simulink model "chap04"  (R2021a)
settings: Solver=FixedStepDiscrete  StartTime=0.0  StopTime=30  FixedStep=0.001  RelTol=1e-3
undefined symbols (not defined in the file): DiscIntNeverNeededParam
libraries: simulink x4
(part 2 of 7)

== system chap04/Subsystem/Subsystem2 ==
  In19 : Inport
  Bus Creator : BusCreator  Inputs=3
  Bus Selector : BusSelector  OutputSignals=state(tk).node2.xx,state(tk).node1.xx,state(tk).node4.xx,state(tk).node6.xx,state(tk).node2.vx,state(tk).node1.vx,state(tk).node4.vx,state(tk).node6.vx
  Bus Selector1 : BusSelector  OutputSignals=state(tk).node2.xy,state(tk).node1.xy,state(tk).node4.xy,state(tk).node6.xy,state(tk).node2.vy,state(tk).node1.vy,state(tk).node4.vy,state(tk).node6.vy
  Bus Selector2 : BusSelector  OutputSignals=state(tk).node2.xz,state(tk).node1.xz,state(tk).node4.xz,state(tk).node6.xz,state(tk).node2.vz,state(tk).node1.vz,state(tk).node4.vz,state(tk).node6.vz
  Bus Selector3 : BusSelector  OutputSignals=state(t).node2.vx
  Bus Selector4 : BusSelector  OutputSignals=state(t).node2.vy
  Bus Selector5 : BusSelector  OutputSignals=state(t).node2.vz
  Bus Selector6 : BusSelector  OutputSignals=state(t).node2.vx,state(t).node2.vy,state(t).node2.vz
  Bus Selector7 : BusSelector  OutputSignals=state(t).node2.vx,state(t).node2.vy,state(t).node2.vz
  Bus Selector8 : BusSelector  OutputSignals=control.node2.ux,control.node2.uy,control.node2.uz
  Subsystem1 : Subsystem
  Subsystem10 : Subsystem
  Subsystem12 : Subsystem
  Subsystem2 : Subsystem
  Subsystem3 : Subsystem
  Subsystem4 : Subsystem
      settings: PortSchema="{\"entries\":[{\"content\":{\"sides\":[{\"content\":{\"connectorIds\":[\"In1\",\"In2\",\"In3\"]},\"type\":\"ConnectorPlacement.EquallySpacedRectSide\",\"uuid\":\"3c32f130-2df4-4697-80e9-267a8217898e\"},{\"content\":{\"connectorIds\":[\"Out1\"],\"side\":\"RIGHT\"},\"type\":\"ConnectorPlacement.EquallySpacedRectSide\",\"uuid\":\"840675a7-4714-440f-a6ce-75eff1b2763f\"},{\"content\":{\"connectorIds\":[],\"side\":\"TOP\"},\"type\":\"ConnectorPlacement.EquallySpacedRectSide\",\"uuid\":\"5c23af56-4ec3-4a39-a531-12998a0be3c8\"},{\"content\":{\"connectorIds\":[\"Out2\"],\"side\":\"BOTTOM\"},\"type\":\"ConnectorPlacement.EquallySpacedRectSide\",\"uuid\":\"31d953fb-65a0-42e9-a844-060de010f298\"}]},\"type\":\"ConnectorPlacement.EquallySpacedConnector\",\"uuid\":\"61b27aa3-5880-401e-bae3-4611093a191a\"}],\"packageUris\":[\"http://schema.mathworks.com/mf0/Connector/R2020b\"],\"version\":\"1.0\"}"
  Subsystem6 : Subsystem
  Subsystem7 : Subsystem
      settings: PortSchema="{\"entries\":[{\"content\":{\"sides\":[{\"content\":{\"connectorIds\":[\"In1\",\"In2\",\"In3\"]},\"type\":\"ConnectorPlacement.EquallySpacedRectSide\",\"uuid\":\"3c32f130-2df4-4697-80e9-267a8217898e\"},{\"content\":{\"connectorIds\":[\"Out1\"],\"side\":\"RIGHT\"},\"type\":\"ConnectorPlacement.EquallySpacedRectSide\",\"uuid\":\"840675a7-4714-440f-a6ce-75eff1b2763f\"},{\"content\":{\"connectorIds\":[],\"side\":\"TOP\"},\"type\":\"ConnectorPlacement.EquallySpacedRectSide\",\"uuid\":\"5c23af56-4ec3-4a39-a531-12998a0be3c8\"},{\"content\":{\"connectorIds\":[\"Out2\"],\"side\":\"BOTTOM\"},\"type\":\"ConnectorPlacement.EquallySpacedRectSide\",\"uuid\":\"31d953fb-65a0-42e9-a844-060de010f298\"}]},\"type\":\"ConnectorPlacement.EquallySpacedConnector\",\"uuid\":\"61b27aa3-5880-401e-bae3-4611093a191a\"}],\"packageUris\":[\"http://schema.mathworks.com/mf0/Connector/R2020b\"],\"version\":\"1.0\"}"
  Subsystem8 : Subsystem
      settings: PortSchema="{\"entries\":[{\"content\":{\"sides\":[{\"content\":{\"connectorIds\":[\"In1\",\"In2\",\"In3\"]},\"type\":\"ConnectorPlacement.EquallySpacedRectSide\",\"uuid\":\"3c32f130-2df4-4697-80e9-267a8217898e\"},{\"content\":{\"connectorIds\":[\"Out1\"],\"side\":\"RIGHT\"},\"type\":\"ConnectorPlacement.EquallySpacedRectSide\",\"uuid\":\"840675a7-4714-440f-a6ce-75eff1b2763f\"},{\"content\":{\"connectorIds\":[],\"side\":\"TOP\"},\"type\":\"ConnectorPlacement.EquallySpacedRectSide\",\"uuid\":\"5c23af56-4ec3-4a39-a531-12998a0be3c8\"},{\"content\":{\"connectorIds\":[\"Out2\"],\"side\":\"BOTTOM\"},\"type\":\"ConnectorPlacement.EquallySpacedRectSide\",\"uuid\":\"31d953fb-65a0-42e9-a844-060de010f298\"}]},\"type\":\"ConnectorPlacement.EquallySpacedConnector\",\"uuid\":\"61b27aa3-5880-401e-bae3-4611093a191a\"}],\"packageUris\":[\"http://schema.mathworks.com/mf0/Connector/R2020b\"],\"version\":\"1.0\"}"
  u2 : Outport
  wires:
  Bus Creator/1 -> u2/1  "node2"
  Bus Selector6/1 -> Subsystem12/4(vx)  "<vx>"
  Bus Selector6/2 -> Subsystem12/5(vy)  "<vy>"
  Bus Selector6/3 -> Subsystem12/6(vz)  "<vz>"
  [Sz] -> Subsystem12/3(Sz)
  [Sx] -> Subsystem12/1(Sx)
  [state] -> Bus Selector6/1
  [Sy] -> Subsystem12/2(Sy)
  Subsystem12/1(" gain") -> [gain]
  Subsystem10/1(ux) -> Bus Creator/1  "ux"
  Subsystem10/2(uy) -> Bus Creator/2  "uy"
  Subsystem10/3(uz) -> Bus Creator/3  "uz"
  Bus Selector8/3 -> Subsystem3/8(uz)  "<uz>"
  Bus Selector7/3 -> Subsystem3/4(vz)  "<vz>"
  Bus Selector7/2 -> Subsystem3/3(vy)  "<vy>"
  Bus Selector7/1 -> Subsystem3/2(vx)  "<vx>"
  Bus Selector8/1 -> Subsystem3/6(ux)  "<ux>"
  [state] -> Bus Selector7/1
  Bus Selector8/2 -> Subsystem3/7(uy)  "<uy>"
  [state] -> Bus Selector8/1
  Subsystem3/1(xdut1) -> Subsystem10/1(utx)
  Subsystem3/2(ydut1) -> Subsystem10/2(uty)
  Subsystem3/3(zdut1) -> Subsystem10/3(utz)
  Subsystem8/2(Sz) -> [Sz]
  Subsystem7/1(ux) -> Subsystem3/5(uty)
  Subsystem1/1(p2y) -> Subsystem7/2(uty)
  [state] -> Bus Selector4/1
  Subsystem4/1(ux) -> Subsystem3/1(utx)
  Subsystem2/1(p2z) -> Subsystem8/2(utz)
  Bus Selector4/1 -> Subsystem7/1(vy1)  "<vy>"
  Bus Selector5/1 -> Subsystem8/1(vz1)  "<vz>"
  [gain] -> Subsystem8/3(gain)
  [gain] -> Subsystem4/3(gain)
  Subsystem8/1(ux) -> Subsystem3/9(utz)
  [gain] -> Subsystem7/3(gain)
  [state] -> Bus Selector3/1
  Subsystem6/1(p2x) -> Subsystem4/2(utx)
  Subsystem7/2(Sy) -> [Sy]
  Bus Selector3/1 -> Subsystem4/1(vx1)  "<vx>"
  Subsystem4/2(Sx) -> [Sx]
  [state] -> Bus Selector5/1
  In19/1 -> [state], Bus Selector2/1, Bus Selector/1, Bus Selector1/1
  Bus Selector1/6 -> Subsystem1/6(vy1)  "<vy>"
  Bus Selector2/6 -> Subsystem2/6(vz1)  "<vz>"
  Bus Selector/7 -> Subsystem6/7(vx4)  "<vx>"
  Bus Selector/3 -> Subsystem6/3(xx4)  "<xx>"
  Bus Selector1/2 -> Subsystem1/2(xy1)  "<xy>"
  Bus Selector1/5 -> Subsystem1/5(vy2)  "<vy>"
  Bus Selector/2 -> Subsystem6/2(xx1)  "<xx>"
  Bus Selector/6 -> Subsystem6/6(vx1)  "<vx>"
  Bus Selector/8 -> Subsystem6/8(vx6)  "<vx>"
  Bus Selector1/8 -> Subsystem1/8(vy6)  "<vy>"
  Bus Selector/1 -> Subsystem6/1(xx2)  "<xx>"
  Bus Selector/5 -> Subsystem6/5(vx2)  "<vx>"
  Bus Selector1/1 -> Subsystem1/1(xy2)  "<xy>"
  Bus Selector2/3 -> Subsystem2/3(xz4)  "<xz>"
  Bus Selector2/4 -> Subsystem2/4(xz6)  "<xz>"
  Bus Selector2/5 -> Subsystem2/5(vz2)  "<vz>"
  Bus Selector2/7 -> Subsystem2/7(vz4)  "<vz>"
  Bus Selector2/1 -> Subsystem2/1(xz2)  "<xz>"
  Bus Selector2/2 -> Subsystem2/2(xz1)  "<xz>"
  Bus Selector1/7 -> Subsystem1/7(vy4)  "<vy>"
  Bus Selector1/3 -> Subsystem1/3(xy4)  "<xy>"
  Bus Selector1/4 -> Subsystem1/4(xy6)  "<xy>"
  Bus Selector/4 -> Subsystem6/4(xx6)  "<xx>"
  Bus Selector2/8 -> Subsystem2/8(vz6)  "<vz>"

== system chap04/Subsystem/Subsystem3 ==
  In19 : Inport
  Bus Creator : BusCreator  Inputs=3
  Bus Selector : BusSelector  OutputSignals=state(tk).node4.xx,state(tk).node2.xx,state(tk).node3.xx,state(tk).node5.xx,state(tk).node4.vx,state(tk).node2.vx,state(tk).node3.vx,state(tk).node5.vx
  Bus Selector1 : BusSelector  OutputSignals=state(tk).node4.xy,state(tk).node2.xy,state(tk).node3.xy,state(tk).node5.xy,state(tk).node4.vy,state(tk).node2.vy,state(tk).node3.vy,state(tk).node5.vy
  Bus Selector2 : BusSelector  OutputSignals=state(tk).node4.xz,state(tk).node2.xz,state(tk).node3.xz,state(tk).node5.xz,state(tk).node4.vz,state(tk).node2.vz,state(tk).node3.vz,state(tk).node5.vz
  Bus Selector3 : BusSelector  OutputSignals=state(t).node4.vx
  Bus Selector4 : BusSelector  OutputSignals=state(t).node4.vy
  Bus Selector5 : BusSelector  OutputSignals=state(t).node4.vz
  Bus Selector6 : BusSelector  OutputSignals=state(t).node4.vx,state(t).node4.vy,state(t).node4.vz
  Bus Selector7 : BusSelector  OutputSignals=state(t).node4.vx,state(t).node4.vy,state(t).node4.vz
  Bus Selector8 : BusSelector  OutputSignals=control.node4.ux,control.node4.uy,control.node4.uz
  Subsystem1 : Subsystem
  Subsystem10 : Subsystem
  Subsystem12 : Subsystem
  Subsystem2 : Subsystem
  Subsystem3 : Subsystem
  Subsystem4 : Subsystem
      settings: PortSchema="{\"entries\":[{\"content\":{\"sides\":[{\"content\":{\"connectorIds\":[\"In1\",\"In2\",\"In3\"]},\"type\":\"ConnectorPlacement.EquallySpacedRectSide\",\"uuid\":\"3c32f130-2df4-4697-80e9-267a8217898e\"},{\"content\":{\"connectorIds\":[\"Out1\"],\"side\":\"RIGHT\"},\"type\":\"ConnectorPlacement.EquallySpacedRectSide\",\"uuid\":\"840675a7-4714-440f-a6ce-75eff1b2763f\"},{\"content\":{\"connectorIds\":[],\"side\":\"TOP\"},\"type\":\"ConnectorPlacement.EquallySpacedRectSide\",\"uuid\":\"5c23af56-4ec3-4a39-a531-12998a0be3c8\"},{\"content\":{\"connectorIds\":[\"Out2\"],\"side\":\"BOTTOM\"},\"type\":\"ConnectorPlacement.EquallySpacedRectSide\",\"uuid\":\"31d953fb-65a0-42e9-a844-060de010f298\"}]},\"type\":\"ConnectorPlacement.EquallySpacedConnector\",\"uuid\":\"61b27aa3-5880-401e-bae3-4611093a191a\"}],\"packageUris\":[\"http://schema.mathworks.com/mf0/Connector/R2020b\"],\"version\":\"1.0\"}"
  Subsystem6 : Subsystem
  Subsystem7 : Subsystem
      settings: PortSchema="{\"entries\":[{\"content\":{\"sides\":[{\"content\":{\"connectorIds\":[\"In1\",\"In2\",\"In3\"]},\"type\":\"ConnectorPlacement.EquallySpacedRectSide\",\"uuid\":\"3c32f130-2df4-4697-80e9-267a8217898e\"},{\"content\":{\"connectorIds\":[\"Out1\"],\"side\":\"RIGHT\"},\"type\":\"ConnectorPlacement.EquallySpacedRectSide\",\"uuid\":\"840675a7-4714-440f-a6ce-75eff1b2763f\"},{\"content\":{\"connectorIds\":[],\"side\":\"TOP\"},\"type\":\"ConnectorPlacement.EquallySpacedRectSide\",\"uuid\":\"5c23af56-4ec3-4a39-a531-12998a0be3c8\"},{\"content\":{\"connectorIds\":[\"Out2\"],\"side\":\"BOTTOM\"},\"type\":\"ConnectorPlacement.EquallySpacedRectSide\",\"uuid\":\"31d953fb-65a0-42e9-a844-060de010f298\"}]},\"type\":\"ConnectorPlacement.EquallySpacedConnector\",\"uuid\":\"61b27aa3-5880-401e-bae3-4611093a191a\"}],\"packageUris\":[\"http://schema.mathworks.com/mf0/Connector/R2020b\"],\"version\":\"1.0\"}"
  Subsystem8 : Subsystem
      settings: PortSchema="{\"entries\":[{\"content\":{\"sides\":[{\"content\":{\"connectorIds\":[\"In1\",\"In2\",\"In3\"]},\"type\":\"ConnectorPlacement.EquallySpacedRectSide\",\"uuid\":\"3c32f130-2df4-4697-80e9-267a8217898e\"},{\"content\":{\"connectorIds\":[\"Out1\"],\"side\":\"RIGHT\"},\"type\":\"ConnectorPlacement.EquallySpacedRectSide\",\"uuid\":\"840675a7-4714-440f-a6ce-75eff1b2763f\"},{\"content\":{\"connectorIds\":[],\"side\":\"TOP\"},\"type\":\"ConnectorPlacement.EquallySpacedRectSide\",\"uuid\":\"5c23af56-4ec3-4a39-a531-12998a0be3c8\"},{\"content\":{\"connectorIds\":[\"Out2\"],\"side\":\"BOTTOM\"},\"type\":\"ConnectorPlacement.EquallySpacedRectSide\",\"uuid\":\"31d953fb-65a0-42e9-a844-060de010f298\"}]},\"type\":\"ConnectorPlacement.EquallySpacedConnector\",\"uuid\":\"61b27aa3-5880-401e-bae3-4611093a191a\"}],\"packageUris\":[\"http://schema.mathworks.com/mf0/Connector/R2020b\"],\"version\":\"1.0\"}"
  u4 : Outport
  wires:
  Bus Creator/1 -> u4/1  "node4"
  Bus Selector/2 -> Subsystem6/2(xx2)  "<xx>"
  Bus Selector1/7 -> Subsystem1/7(vy3)  "<vy>"
  Bus Selector1/4 -> Subsystem1/4(xy5)  "<xy>"
  Bus Selector2/3 -> Subsystem2/3(xz3)  "<xz>"
  Bus Selector/8 -> Subsystem6/8(vx5)  "<vx>"
  Bus Selector2/2 -> Subsystem2/2(xx2)  "<xz>"
  Bus Selector2/4 -> Subsystem2/4(xz5)  "<xz>"
  Bus Selector1/5 -> Subsystem1/5(vy4)  "<vy>"
  Bus Selector1/2 -> Subsystem1/2(xy2)  "<xy>"
  Bus Selector2/7 -> Subsystem2/7(vz3)  "<vz>"
  Bus Selector2/5 -> Subsystem2/5(vz4)  "<vz>"
  Bus Selector1/6 -> Subsystem1/6(vy2)  "<vy>"
  Bus Selector2/8 -> Subsystem2/8(vz5)  "<vz>"
  Bus Selector2/6 -> Subsystem2/6(vz2)  "<vz>"
  Bus Selector1/3 -> Subsystem1/3(xy3)  "<xy>"
  Bus Selector2/1 -> Subsystem2/1(xz4)  "<xz>"
  Bus Selector/5 -> Subsystem6/5(vx4)  "<vx>"
  Bus Selector/1 -> Subsystem6/1(xx4)  "<xx>"
  Bus Selector/3 -> Subsystem6/3(xx3)  "<xx>"
  Bus Selector1/8 -> Subsystem1/8(vy5)  "<vy>"
  Bus Selector1/1 -> Subsystem1/1(xy4)  "<xy>"
  Bus Selector/7 -> Subsystem6/7(vx3)  "<vx>"
  Bus Selector/6 -> Subsystem6/6(vx2)  "<vx>"
  Bus Selector/4 -> Subsystem6/4(xx5)  "<xx>"
  [state] -> Bus Selector5/1
  Subsystem2/1(utx) -> Subsystem8/2(utz)
  Bus Selector5/1 -> Subsystem8/1(vz4)  "<vz>"
  [state] -> Bus Selector4/1
  [gain] -> Subsystem8/3(gain)
  Bus Selector6/3 -> Subsystem12/6(vz)  "<vz>"
  Bus Selector6/1 -> Subsystem12/4(vx)  "<vx>"
  [Sx] -> Subsystem12/1(Sx)
  [Sz] -> Subsystem12/3(Sz)
  Subsystem12/1(" gain") -> [gain]
  Subsystem6/1(utx) -> Subsystem4/2(utx)
  In19/1 -> [state], Bus Selector2/1, Bus Selector/1, Bus Selector1/1
  [state] -> Bus Selector6/1
  Bus Selector4/1 -> Subsystem7/1(vy4)  "<vy>"
  Subsystem1/1(utx) -> Subsystem7/2(uty)
  Bus Selector3/1 -> Subsystem4/1(vx4)  "<vx>"
  Subsystem7/2(Sy) -> [Sy]
  [gain] -> Subsystem7/3(gain)
  [Sy] -> Subsystem12/2(Sy)
  [gain] -> Subsystem4/3(gain)
  [state] -> Bus Selector3/1
  Subsystem8/2(Sz) -> [Sz]
  Bus Selector6/2 -> Subsystem12/5(vy)  "<vy>"
  Subsystem4/2(Sx) -> [Sx]
  Subsystem10/1(ux) -> Bus Creator/1  "ux"
  Subsystem10/2(uy) -> Bus Creator/2  "uy"
  Subsystem10/3(uz) -> Bus Creator/3  "uz"
  Subsystem4/1(ux) -> Subsystem3/1(utx)
  Subsystem7/1(ux) -> Subsystem3/5(uty)
  Subsystem8/1(ux) -> Subsystem3/9(utz)
  [state] -> Bus Selector7/1
  Bus Selector8/1 -> Subsystem3/6(ux)  "<ux>"
  Bus Selector7/2 -> Subsystem3/3(vy)  "<vy>"
  Bus Selector8/2 -> Subsystem3/7(uy)  "<uy>"
  [state] -> Bus Selector8/1
  Bus Selector7/1 -> Subsystem3/2(vx)  "<vx>"
  Bus Selector7/3 -> Subsystem3/4(vz)  "<vz>"
  Bus Selector8/3 -> Subsystem3/8(uz)  "<uz>"
  Subsystem3/1(udtx) -> Subsystem10/1(utx)
  Subsystem3/2(udty) -> Subsystem10/2(uty)
  Subsystem3/3(udtz) -> Subsystem10/3(utz)

== system chap04/Subsystem/Subsystem4 ==
  In19 : Inport
  Bus Creator : BusCreator  Inputs=3
  Bus Selector : BusSelector  OutputSignals=state(tk).node6.xx,state(tk).node6.xx0,state(tk).node1.xx,state(tk).node2.xx,state(tk).node6.vx,state(tk).node6.vx0,state(tk).node1.vx,state(tk).node2.vx
  Bus Selector1 : BusSelector  OutputSignals=state(tk).node6.xy,state(tk).node6.xy0,state(tk).node1.xy,state(tk).node2.xy,state(tk).node6.vy,state(tk).node6.vy0,state(tk).node1.vy,state(tk).node2.vy
  Bus Selector2 : BusSelector  OutputSignals=state(tk).node6.xz,state(tk).node6.xz0,state(tk).node1.xz,state(tk).node2.xz,state(tk).node6.vz,state(tk).node6.vz0,state(tk).node1.vz,state(tk).node2.vz
  Bus Selector3 : BusSelector  OutputSignals=state(t).node6.vx,state(t).node0.vx
  Bus Selector4 : BusSelector  OutputSignals=state(t).node6.vy,state(t).node0.vx
  Bus Selector5 : BusSelector  OutputSignals=state(t).node6.vz,state(t).node0.vz
  Bus Selector6 : BusSelector  OutputSignals=state(t).node6.vx,state(t).node6.vy,state(t).node6.vz
  Bus Selector7 : BusSelector  OutputSignals=state(t).node6.vx,state(t).node6.vy,state(t).node6.vz
  Bus Selector8 : BusSelector  OutputSignals=control.node6.ux,control.node6.uy,control.node6.uz
  Subsystem1 : Subsystem
  Subsystem10 : Subsystem
  Subsystem12 : Subsystem
  Subsystem2 : Subsystem
  Subsystem3 : Subsystem
  Subsystem4 : Subsystem
      settings: PortSchema="{\"entries\":[{\"content\":{\"sides\":[{\"content\":{\"connectorIds\":[\"In1\",\"In2\",\"In3\",\"In4\"]},\"type\":\"ConnectorPlacement.EquallySpacedRectSide\",\"uuid\":\"3c32f130-2df4-4697-80e9-267a8217898e\"},{\"content\":{\"connectorIds\":[\"Out1\"],\"side\":\"RIGHT\"},\"type\":\"ConnectorPlacement.EquallySpacedRectSide\",\"uuid\":\"840675a7-4714-440f-a6ce-75eff1b2763f\"},{\"content\":{\"connectorIds\":[],\"side\":\"TOP\"},\"type\":\"ConnectorPlacement.EquallySpacedRectSide\",\"uuid\":\"5c23af56-4ec3-4a39-a531-12998a0be3c8\"},{\"content\":{\"connectorIds\":[\"Out2\"],\"side\":\"BOTTOM\"},\"type\":\"ConnectorPlacement.EquallySpacedRectSide\",\"uuid\":\"31d953fb-65a0-42e9-a844-060de010f298\"}]},\"type\":\"ConnectorPlacement.EquallySpacedConnector\",\"uuid\":\"61b27aa3-5880-401e-bae3-4611093a191a\"}],\"packageUris\":[\"http://schema.mathworks.com/mf0/Connector/R2020b\"],\"version\":\"1.0\"}"
  Subsystem6 : Subsystem
  Subsystem7 : Subsystem
      settings: PortSchema="{\"entries\":[{\"content\":{\"sides\":[{\"content\":{\"connectorIds\":[\"In1\",\"In2\",\"In3\",\"In4\"]},\"type\":\"ConnectorPlacement.EquallySpacedRectSide\",\"uuid\":\"3c32f130-2df4-4697-80e9-267a8217898e\"},{\"content\":{\"connectorIds\":[\"Out1\"],\"side\":\"RIGHT\"},\"type\":\"ConnectorPlacement.EquallySpacedRectSide\",\"uuid\":\"840675a7-4714-440f-a6ce-75eff1b2763f\"},{\"content\":{\"connectorIds\":[],\"side\":\"TOP\"},\"type\":\"ConnectorPlacement.EquallySpacedRectSide\",\"uuid\":\"5c23af56-4ec3-4a39-a531-12998a0be3c8\"},{\"content\":{\"connectorIds\":[\"Out2\"],\"side\":\"BOTTOM\"},\"type\":\"ConnectorPlacement.EquallySpacedRectSide\",\"uuid\":\"31d953fb-65a0-42e9-a844-060de010f298\"}]},\"type\":\"ConnectorPlacement.EquallySpacedConnector\",\"uuid\":\"61b27aa3-5880-401e-bae3-4611093a191a\"}],\"packageUris\":[\"http://schema.mathworks.com/mf0/Connector/R2020b\"],\"version\":\"1.0\"}"
  Subsystem8 : Subsystem
      settings: PortSchema="{\"entries\":[{\"content\":{\"sides\":[{\"content\":{\"connectorIds\":[\"In1\",\"In2\",\"In3\",\"In4\"]},\"type\":\"ConnectorPlacement.EquallySpacedRectSide\",\"uuid\":\"3c32f130-2df4-4697-80e9-267a8217898e\"},{\"content\":{\"connectorIds\":[\"Out1\"],\"side\":\"RIGHT\"},\"type\":\"ConnectorPlacement.EquallySpacedRectSide\",\"uuid\":\"840675a7-4714-440f-a6ce-75eff1b2763f\"},{\"content\":{\"connectorIds\":[],\"side\":\"TOP\"},\"type\":\"ConnectorPlacement.EquallySpacedRectSide\",\"uuid\":\"5c23af56-4ec3-4a39-a531-12998a0be3c8\"},{\"content\":{\"connectorIds\":[\"Out2\"],\"side\":\"BOTTOM\"},\"type\":\"ConnectorPlacement.EquallySpacedRectSide\",\"uuid\":\"31d953fb-65a0-42e9-a844-060de010f298\"}]},\"type\":\"ConnectorPlacement.EquallySpacedConnector\",\"uuid\":\"61b27aa3-5880-401e-bae3-4611093a191a\"}],\"packageUris\":[\"http://schema.mathworks.com/mf0/Connector/R2020b\"],\"version\":\"1.0\"}"
  u6 : Outport
  wires:
  Bus Creator/1 -> u6/1  "node6"
  Bus Selector/1 -> Subsystem6/1(xx6)  "<xx>"
  Bus Selector/3 -> Subsystem6/3(xx1)  "<xx>"
  Bus Selector/4 -> Subsystem6/4(xx2)  "<xx>"
  Bus Selector6/3 -> Subsystem12/6(vz)  "<vz>"
  Bus Selector6/1 -> Subsystem12/4(vx)  "<vx>"
  [Sx] -> Subsystem12/1(Sx)
  [Sz] -> Subsystem12/3(Sz)
  Subsystem12/1(" gain") -> [gain]
  In19/1 -> [state], Bus Selector2/1, Bus Selector/1, Bus Selector1/1
  [state] -> Bus Selector6/1
  [Sy] -> Subsystem12/2(Sy)
  Bus Selector6/2 -> Subsystem12/5(vy)  "<vy>"
  Subsystem10/3(uz) -> Bus Creator/3  "uz"
  Subsystem10/2(uy) -> Bus Creator/2  "uy"
  Subsystem10/1(ux) -> Bus Creator/1  "ux"
  Bus Selector7/3 -> Subsystem3/4(vz)  "<vz>"
  Bus Selector7/1 -> Subsystem3/2(vx)  "<vx>"
  [state] -> Bus Selector8/1
  Bus Selector8/1 -> Subsystem3/6(ux)  "<ux>"
  Bus Selector8/2 -> Subsystem3/7(uy)  "<uy>"
  Bus Selector7/2 -> Subsystem3/3(vy)  "<vy>"
  [state] -> Bus Selector7/1
  Bus Selector8/3 -> Subsystem3/8(uz)  "<uz>"
  Subsystem3/2(udty) -> Subsystem10/2(uty)
  Subsystem3/1(udtx) -> Subsystem10/1(utx)
  Subsystem3/3(udtz) -> Subsystem10/3(utz)
  Bus Selector/2 -> Subsystem6/2(xx0)  "<xx0>"
  Bus Selector/5 -> Subsystem6/5(vx6)  "<vx>"
  Bus Selector/6 -> Subsystem6/6(vx0)  "<vx0>"
  Bus Selector/7 -> Subsystem6/7(vx1)  "<vx>"
  Bus Selector/8 -> Subsystem6/8(vx2)  "<vx>"
  Bus Selector1/1 -> Subsystem1/1(xx6)  "<xy>"
  Bus Selector1/2 -> Subsystem1/2(xx0)  "<xy0>"
  Bus Selector1/3 -> Subsystem1/3(xx1)  "<xy>"
  Bus Selector1/4 -> Subsystem1/4(xx2)  "<xy>"
  Bus Selector1/5 -> Subsystem1/5(vx6)  "<vy>"
  Bus Selector1/6 -> Subsystem1/6(vx0)  "<vy0>"
  Bus Selector1/7 -> Subsystem1/7(vx1)  "<vy>"
  Bus Selector1/8 -> Subsystem1/8(vx2)  "<vy>"
  Bus Selector2/1 -> Subsystem2/1(xx6)  "<xz>"
  Bus Selector2/2 -> Subsystem2/2(xx0)  "<xz0>"
  Bus Selector2/3 -> Subsystem2/3(xx1)  "<xz>"
  Bus Selector2/4 -> Subsystem2/4(xx2)  "<xz>"
  Bus Selector2/5 -> Subsystem2/5(vx6)  "<vz>"
  Bus Selector2/6 -> Subsystem2/6(vx0)  "<vz0>"
  Bus Selector2/7 -> Subsystem2/7(vx1)  "<vz>"
  Bus Selector2/8 -> Subsystem2/8(vx2)  "<vz>"
  Subsystem4/2(Sx) -> [Sx]
  Bus Selector5/2 -> Subsystem8/2(vz0)  "<vz>"
  Subsystem7/2(Sy) -> [Sy]
  Subsystem8/2(Sz) -> [Sz]
  [gain] -> Subsystem7/4(gain)
  Subsystem1/1(utx) -> Subsystem7/3(uty)
  Subsystem2/1(utx) -> Subsystem8/3(utz)
  [state] -> Bus Selector3/1
  Bus Selector5/1 -> Subsystem8/1(vz6)  "<vz>"
  Bus Selector4/2 -> Subsystem7/2(vy0)  "<vx>"
  [gain] -> Subsystem4/4(gain)
  [state] -> Bus Selector5/1
  Subsystem8/1(ux) -> Subsystem3/9(utz)
  Subsystem6/1(utx) -> Subsystem4/3(utx)
  Subsystem7/1(ux) -> Subsystem3/5(uty)
  Subsystem4/1(ux) -> Subsystem3/1(utx)
  Bus Selector3/1 -> Subsystem4/1(vx6)  "<vx>"
  Bus Selector3/2 -> Subsystem4/2(vx0)  "<vx>"
  [gain] -> Subsystem8/4(gain)
  [state] -> Bus Selector4/1
  Bus Selector4/1 -> Subsystem7/1(vy6)  "<vy>"

== system chap04/Subsystem/Subsystem5 ==
  In19 : Inport
  Bus Creator : BusCreator  Inputs=3
  Bus Selector : BusSelector  OutputSignals=state(tk).node3.xx,state(tk).node1.xx,state(tk).node4.xx,state(tk).node5.xx,state(tk).node3.vx,state(tk).node1.vx,state(tk).node4.vx,state(tk).node5.vx
  Bus Selector1 : BusSelector  OutputSignals=state(tk).node3.xy,state(tk).node1.xy,state(tk).node4.xy,state(tk).node5.xy,state(tk).node3.vy,state(tk).node1.vy,state(tk).node4.vy,state(tk).node5.vy
  Bus Selector2 : BusSelector  OutputSignals=state(tk).node3.xz,state(tk).node1.xz,state(tk).node4.xz,state(tk).node5.xz,state(tk).node3.vz,state(tk).node1.vz,state(tk).node4.vz,state(tk).node5.vz
  Bus Selector3 : BusSelector  OutputSignals=state(t).node3.vx
  Bus Selector4 : BusSelector  OutputSignals=state(t).node3.vy
  Bus Selector5 : BusSelector  OutputSignals=state(t).node3.vz
  Bus Selector6 : BusSelector  OutputSignals=state(t).node3.vx,state(t).node3.vy,state(t).node3.vz
  Bus Selector7 : BusSelector  OutputSignals=state(t).node3.vx,state(t).node3.vy,state(t).node3.vz
  Bus Selector8 : BusSelector  OutputSignals=control.node3.ux,control.node3.uy,control.node3.uz
  Subsystem1 : Subsystem
  Subsystem10 : Subsystem
  Subsystem12 : Subsystem
  Subsystem2 : Subsystem
  Subsystem3 : Subsystem
  Subsystem4 : Subsystem
      settings: PortSchema="{\"entries\":[{\"content\":{\"sides\":[{\"content\":{\"connectorIds\":[\"In1\",\"In2\",\"In3\"]},\"type\":\"ConnectorPlacement.EquallySpacedRectSide\",\"uuid\":\"3c32f130-2df4-4697-80e9-267a8217898e\"},{\"content\":{\"connectorIds\":[\"Out1\"],\"side\":\"RIGHT\"},\"type\":\"ConnectorPlacement.EquallySpacedRectSide\",\"uuid\":\"840675a7-4714-440f-a6ce-75eff1b2763f\"},{\"content\":{\"connectorIds\":[],\"side\":\"TOP\"},\"type\":\"ConnectorPlacement.EquallySpacedRectSide\",\"uuid\":\"5c23af56-4ec3-4a39-a531-12998a0be3c8\"},{\"content\":{\"connectorIds\":[\"Out2\"],\"side\":\"BOTTOM\"},\"type\":\"ConnectorPlacement.EquallySpacedRectSide\",\"uuid\":\"31d953fb-65a0-42e9-a844-060de010f298\"}]},\"type\":\"ConnectorPlacement.EquallySpacedConnector\",\"uuid\":\"61b27aa3-5880-401e-bae3-4611093a191a\"}],\"packageUris\":[\"http://schema.mathworks.com/mf0/Connector/R2020b\"],\"version\":\"1.0\"}"
  Subsystem6 : Subsystem
  Subsystem7 : Subsystem
      settings: PortSchema="{\"entries\":[{\"content\":{\"sides\":[{\"content\":{\"connectorIds\":[\"In1\",\"In2\",\"In3\"]},\"type\":\"ConnectorPlacement.EquallySpacedRectSide\",\"uuid\":\"3c32f130-2df4-4697-80e9-267a8217898e\"},{\"content\":{\"connectorIds\":[\"Out1\"],\"side\":\"RIGHT\"},\"type\":\"ConnectorPlacement.EquallySpacedRectSide\",\"uuid\":\"840675a7-4714-440f-a6ce-75eff1b2763f\"},{\"content\":{\"connectorIds\":[],\"side\":\"TOP\"},\"type\":\"ConnectorPlacement.EquallySpacedRectSide\",\"uuid\":\"5c23af56-4ec3-4a39-a531-12998a0be3c8\"},{\"content\":{\"connectorIds\":[\"Out2\"],\"side\":\"BOTTOM\"},\"type\":\"ConnectorPlacement.EquallySpacedRectSide\",\"uuid\":\"31d953fb-65a0-42e9-a844-060de010f298\"}]},\"type\":\"ConnectorPlacement.EquallySpacedConnector\",\"uuid\":\"61b27aa3-5880-401e-bae3-4611093a191a\"}],\"packageUris\":[\"http://schema.mathworks.com/mf0/Connector/R2020b\"],\"version\":\"1.0\"}"
  Subsystem8 : Subsystem
      settings: PortSchema="{\"entries\":[{\"content\":{\"sides\":[{\"content\":{\"connectorIds\":[\"In1\",\"In2\",\"In3\"]},\"type\":\"ConnectorPlacement.EquallySpacedRectSide\",\"uuid\":\"3c32f130-2df4-4697-80e9-267a8217898e\"},{\"content\":{\"connectorIds\":[\"Out1\"],\"side\":\"RIGHT\"},\"type\":\"ConnectorPlacement.EquallySpacedRectSide\",\"uuid\":\"840675a7-4714-440f-a6ce-75eff1b2763f\"},{\"content\":{\"connectorIds\":[],\"side\":\"TOP\"},\"type\":\"ConnectorPlacement.EquallySpacedRectSide\",\"uuid\":\"5c23af56-4ec3-4a39-a531-12998a0be3c8\"},{\"content\":{\"connectorIds\":[\"Out2\"],\"side\":\"BOTTOM\"},\"type\":\"ConnectorPlacement.EquallySpacedRectSide\",\"uuid\":\"31d953fb-65a0-42e9-a844-060de010f298\"}]},\"type\":\"ConnectorPlacement.EquallySpacedConnector\",\"uuid\":\"61b27aa3-5880-401e-bae3-4611093a191a\"}],\"packageUris\":[\"http://schema.mathworks.com/mf0/Connector/R2020b\"],\"version\":\"1.0\"}"
  u3 : Outport
  wires:
  Bus Creator/1 -> u3/1  "node3"
  [state] -> Bus Selector6/1
  [Sz] -> Subsystem12/3(Sz)
  [Sx] -> Subsystem12/1(Sx)
  Bus Selector6/3 -> Subsystem12/6(vz)  "<vz>"
  [Sy] -> Subsystem12/2(Sy)
  Bus Selector6/1 -> Subsystem12/4(vx)  "<vx>"
  Bus Selector6/2 -> Subsystem12/5(vy)  "<vy>"
  Subsystem10/1(ux) -> Bus Creator/1  "ux"
  Subsystem10/2(uy) -> Bus Creator/2  "uy"
  Subsystem10/3(uz) -> Bus Creator/3  "uz"
  [state] -> Bus Selector7/1
  Bus Selector8/1 -> Subsystem3/6(ux)  "<ux>"
  Bus Selector7/2 -> Subsystem3/3(vy)  "<vy>"
  Bus Selector8/2 -> Subsystem3/7(uy)  "<uy>"
  [state] -> Bus Selector8/1
  Bus Selector7/1 -> Subsystem3/2(vx)  "<vx>"
  Bus Selector7/3 -> Subsystem3/4(vz)  "<vz>"
  Bus Selector8/3 -> Subsystem3/8(uz)  "<uz>"
  Subsystem3/1(udtx) -> Subsystem10/1(utx)
  Subsystem3/2(udty) -> Subsystem10/2(uty)
  Subsystem3/3(udtz) -> Subsystem10/3(utz)
  Subsystem12/1(" gain") -> [gain]
  Bus Selector2/8 -> Subsystem2/8(vz5)  "<vz>"
  In19/1 -> Bus Selector/1, Bus Selector1/1, [state], Bus Selector2/1
  Bus Selector1/4 -> Subsystem1/4(xy5)  "<xy>"
  Bus Selector/4 -> Subsystem6/4(xx5)  "<xx>"
  Bus Selector/2 -> Subsystem6/2(xx1)  "<xx>"
  Bus Selector/1 -> Subsystem6/1(xx3)  "<xx>"
  Bus Selector/8 -> Subsystem6/8(vx5)  "<vx>"
  Bus Selector2/7 -> Subsystem2/7(vz4)  "<vz>"
  Bus Selector1/5 -> Subsystem1/5(vy3)  "<vy>"
  Bus Selector1/1 -> Subsystem1/1(xy3)  "<xy>"
  Bus Selector/3 -> Subsystem6/3(xx4)  "<xx>"
  Bus Selector/5 -> Subsystem6/5(vx3)  "<vx>"
  Bus Selector1/6 -> Subsystem1/6(vy1)  "<vy>"
  Bus Selector2/3 -> Subsystem2/3(xz4)  "<xz>"
  Bus Selector1/8 -> Subsystem1/8(vy5)  "<vy>"
  Bus Selector2/1 -> Subsystem2/1(xz3)  "<xz>"
  Bus Selector1/3 -> Subsystem1/3(xy4)  "<xy>"
  Bus Selector1/2 -> Subsystem1/2(xy1)  "<xy>"
  Bus Selector1/7 -> Subsystem1/7(vy4)  "<vy>"
  Bus Selector2/2 -> Subsystem2/2(xz1)  "<xz>"
  Bus Selector2/4 -> Subsystem2/4(xz5)  "<xz>"
  Bus Selector2/6 -> Subsystem2/6(vz1)  "<vz>"
  Bus Selector2/5 -> Subsystem2/5(vz3)  "<vz>"
  Bus Selector/7 -> Subsystem6/7(vx4)  "<vx>"
  Bus Selector/6 -> Subsystem6/6(vx1)  "<vx>"
  Subsystem6/1(p3x) -> Subsystem4/2(utx)
  [gain] -> Subsystem7/3(gain)
  Bus Selector4/1 -> Subsystem7/1(vy3)  "<vy>"
  [state] -> Bus Selector5/1
  [state] -> Bus Selector3/1
  Subsystem4/2(Sx) -> [Sx]
  Bus Selector3/1 -> Subsystem4/1(vx3)  "<vx>"
  Subsystem7/1(ux) -> Subsystem3/5(uty)
  Bus Selector5/1 -> Subsystem8/1(vz3)  "<vz>"
  [gain] -> Subsystem4/3(gain)
  Subsystem8/1(ux) -> Subsystem3/9(utz)
  [gain] -> Subsystem8/3(gain)
  Subsystem2/1(p3z) -> Subsystem8/2(utz)
  Subsystem4/1(ux) -> Subsystem3/1(utx)
  Subsystem1/1(p3y) -> Subsystem7/2(uty)
  [state] -> Bus Selector4/1
  Subsystem8/2(Sz) -> [Sz]
  Subsystem7/2(Sy) -> [Sy]

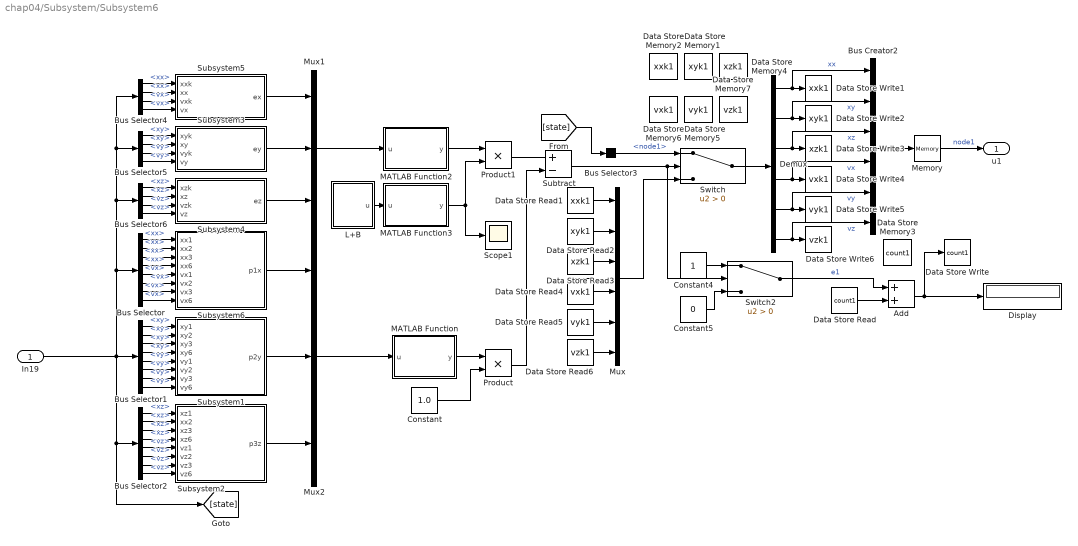
== system chap04/Subsystem/Subsystem6 ==
  In19 : Inport
  Add : Sum
  Bus Creator2 : BusCreator  Inputs=6
  Bus Selector : BusSelector  OutputSignals=state(tk).node1.xx,state(tk).node2.xx,state(tk).node3.xx,state(tk).node6.xx,state(tk).node1.vx,state(tk).node2.vx,state(tk).node3.vx,state(tk).node6.vx
  Bus Selector1 : BusSelector  OutputSignals=state(tk).node1.xy,state(tk).node2.xy,state(tk).node3.xy,state(tk).node6.xy,state(tk).node1.vy,state(tk).node2.vy,state(tk).node3.vy,state(tk).node6.vy
  Bus Selector2 : BusSelector  OutputSignals=state(tk).node1.xz,state(tk).node2.xz,state(tk).node3.xz,state(tk).node6.xz,state(tk).node1.vz,state(tk).node2.vz,state(tk).node3.vz,state(tk).node6.vz
  Bus Selector3 : BusSelector  OutputSignals=state(t).node1
  Bus Selector4 : BusSelector  OutputSignals=state(tk).node1.xx,state(t).node1.xx,state(tk).node1.vx,state(t).node1.vx
  Bus Selector5 : BusSelector  OutputSignals=state(tk).node1.xy,state(t).node1.xy,state(tk).node1.vy,state(t).node1.vy
  Bus Selector6 : BusSelector  OutputSignals=state(tk).node1.xz,state(t).node1.xz,state(tk).node1.vz,state(t).node1.vz
  Constant : Constant  Value=1.0
  Constant4 : Constant
  Constant5 : Constant  Value=0
  Data Store Memory1 : DataStoreMemory  DataStoreName=xyk1  ReadBeforeWriteMsg=warning  WriteAfterWriteMsg=warning  WriteAfterReadMsg=warning  ShowAdditionalParam=off
  Data Store Memory2 : DataStoreMemory  DataStoreName=xxk1  ReadBeforeWriteMsg=warning  WriteAfterWriteMsg=warning  WriteAfterReadMsg=warning  ShowAdditionalParam=off
  Data Store Memory3 : DataStoreMemory  DataStoreName=count1  ReadBeforeWriteMsg=warning  WriteAfterWriteMsg=warning  WriteAfterReadMsg=warning  ShowAdditionalParam=off
  Data Store Memory4 : DataStoreMemory  DataStoreName=xzk1  ReadBeforeWriteMsg=warning  WriteAfterWriteMsg=warning  WriteAfterReadMsg=warning  ShowAdditionalParam=off
  Data Store Memory5 : DataStoreMemory  DataStoreName=vyk1  ReadBeforeWriteMsg=warning  WriteAfterWriteMsg=warning  WriteAfterReadMsg=warning  ShowAdditionalParam=off
  Data Store Memory6 : DataStoreMemory  DataStoreName=vxk1  ReadBeforeWriteMsg=warning  WriteAfterWriteMsg=warning  WriteAfterReadMsg=warning  ShowAdditionalParam=off
  Data Store Memory7 : DataStoreMemory  DataStoreName=vzk1  ReadBeforeWriteMsg=warning  WriteAfterWriteMsg=warning  WriteAfterReadMsg=warning  ShowAdditionalParam=off
  Data Store Read : DataStoreRead  DataStoreName=count1  IndexOptions=Index vector (dialog)  Indices=1  OutputSizes=1
  Data Store Read1 : DataStoreRead  DataStoreName=xxk1  IndexOptions=Index vector (dialog)  Indices=1  OutputSizes=1
  Data Store Read2 : DataStoreRead  DataStoreName=xyk1  IndexOptions=Index vector (dialog)  Indices=1  OutputSizes=1
  Data Store Read3 : DataStoreRead  DataStoreName=xzk1  IndexOptions=Index vector (dialog)  Indices=1  OutputSizes=1
  Data Store Read4 : DataStoreRead  DataStoreName=vxk1  IndexOptions=Index vector (dialog)  Indices=1  OutputSizes=1
  Data Store Read5 : DataStoreRead  DataStoreName=vyk1  IndexOptions=Index vector (dialog)  Indices=1  OutputSizes=1
  Data Store Read6 : DataStoreRead  DataStoreName=vzk1  IndexOptions=Index vector (dialog)  Indices=1  OutputSizes=1
  Data Store Write : DataStoreWrite  DataStoreName=count1  IndexOptions=Index vector (dialog)  Indices=1  OutputSizes=1
  Data Store Write1 : DataStoreWrite  DataStoreName=xxk1  IndexOptions=Index vector (dialog)  Indices=1  OutputSizes=1
  Data Store Write2 : DataStoreWrite  DataStoreName=xyk1  IndexOptions=Index vector (dialog)  Indices=1  OutputSizes=1
  Data Store Write3 : DataStoreWrite  DataStoreName=xzk1  IndexOptions=Index vector (dialog)  Indices=1  OutputSizes=1
  Data Store Write4 : DataStoreWrite  DataStoreName=vxk1  IndexOptions=Index vector (dialog)  Indices=1  OutputSizes=1
  Data Store Write5 : DataStoreWrite  DataStoreName=vyk1  IndexOptions=Index vector (dialog)  Indices=1  OutputSizes=1
  Data Store Write6 : DataStoreWrite  DataStoreName=vzk1  IndexOptions=Index vector (dialog)  Indices=1  OutputSizes=1
  Demux : Demux  Outputs=6
  Display : Display
  L+B : Subsystem
  MATLAB Function : MATLAB Function  TreatAsAtomicUnit=on
  MATLAB Function2 : MATLAB Function  TreatAsAtomicUnit=on
  MATLAB Function3 : MATLAB Function  TreatAsAtomicUnit=on
  Memory : Memory
  Mux : Mux  Inputs=6
  Mux1 : Mux  Inputs=3
  Mux2 : Mux  Inputs=3
  Product : Product
  Product1 : Product
  Scope1 : Scope
  Subsystem1 : Subsystem
  Subsystem2 : Subsystem
  Subsystem3 : Subsystem
  Subsystem4 : Subsystem
  Subsystem5 : Subsystem
  Subsystem6 : Subsystem
  Subtract : Sum  Inputs=+-
  Switch : Switch  Criteria=u2 > Threshold
  Switch2 : Switch  Criteria=u2 > Threshold
  u1 : Outport
  wires:
  Bus Selector2/8 -> Subsystem2/8(vz6)  "<vz>"
  Bus Selector2/7 -> Subsystem2/7(vz3)  "<vz>"
  Bus Selector2/6 -> Subsystem2/6(vz2)  "<vz>"
  Bus Selector2/5 -> Subsystem2/5(vz1)  "<vz>"
  Bus Selector2/4 -> Subsystem2/4(xz6)  "<xz>"
  Bus Selector2/3 -> Subsystem2/3(xz3)  "<xz>"
  Bus Selector2/2 -> Subsystem2/2(xx2)  "<xz>"
  Bus Selector2/1 -> Subsystem2/1(xz1)  "<xz>"
  Bus Selector1/8 -> Subsystem1/8(vy6)  "<vy>"
  Bus Selector1/7 -> Subsystem1/7(vy3)  "<vy>"
  Bus Selector1/6 -> Subsystem1/6(vy2)  "<vy>"
  Bus Selector1/5 -> Subsystem1/5(vy1)  "<vy>"
  Bus Selector1/4 -> Subsystem1/4(xy6)  "<xy>"
  Bus Selector1/3 -> Subsystem1/3(xy3)  "<xy>"
  Bus Selector1/2 -> Subsystem1/2(xy2)  "<xy>"
  Bus Selector1/1 -> Subsystem1/1(xy1)  "<xy>"
  Bus Selector/8 -> Subsystem6/8(vx6)  "<vx>"
  Bus Selector/7 -> Subsystem6/7(vx3)  "<vx>"
  Bus Selector/6 -> Subsystem6/6(vx2)  "<vx>"
  Bus Selector/5 -> Subsystem6/5(vx1)  "<vx>"
  Bus Selector/4 -> Subsystem6/4(xx6)  "<xx>"
  Bus Selector/3 -> Subsystem6/3(xx3)  "<xx>"
  Bus Selector/2 -> Subsystem6/2(xx2)  "<xx>"
  Bus Selector/1 -> Subsystem6/1(xx1)  "<xx>"
  Mux2/1 -> MATLAB Function/1(u)
  Subsystem1/1(p2y) -> Mux2/2
  Subsystem6/1(p1x) -> Mux2/1
  Subsystem2/1(p3z) -> Mux2/3
  MATLAB Function/1(y) -> Product/1
  Constant/1 -> Product/2
  Subsystem4/1(ez) -> Mux1/3
  Subsystem5/1(ex) -> Mux1/1
  Subsystem3/1(ey) -> Mux1/2
  Mux1/1 -> MATLAB Function2/1(u)
  MATLAB Function2/1(y) -> Product1/1
  MATLAB Function3/1(y) -> Product1/2, Scope1/1
  Memory/1 -> u1/1  "node1"
  Data Store Read5/1 -> Mux/5
  Data Store Read/1 -> Add/2
  Product1/1 -> Subtract/1
  Add/1 -> Display/1, Data Store Write/1
  Mux/1 -> Switch/3
  Constant4/1 -> Switch2/1
  Data Store Read3/1 -> Mux/3
  Data Store Read1/1 -> Mux/1
  Bus Selector3/1 -> Switch/1  "<node1>"
  Constant5/1 -> Switch2/3
  Switch2/1 -> Add/1  "e1"
  Data Store Read6/1 -> Mux/6
  Switch/1 -> Demux/1
  Data Store Read2/1 -> Mux/2
  Data Store Read4/1 -> Mux/4
  Product/1 -> Subtract/2
  [state] -> Bus Selector3/1
  Demux/1 -> Bus Creator2/1, Data Store Write1/1  "xx"
  Demux/2 -> Bus Creator2/2, Data Store Write2/1  "xy"
  Demux/3 -> Bus Creator2/3, Data Store Write3/1  "xz"
  Demux/4 -> Bus Creator2/4, Data Store Write4/1  "vx"
  Demux/5 -> Bus Creator2/5, Data Store Write5/1  "vy"
  Demux/6 -> Bus Creator2/6, Data Store Write6/1  "vz"
  In19/1 -> [state], Bus Selector2/1, Bus Selector/1, Bus Selector6/1, Bus Selector5/1, Bus Selector4/1, Bus Selector1/1
  Bus Selector6/1 -> Subsystem4/1(xzk)  "<xz>"
  Bus Selector6/2 -> Subsystem4/2(xz)  "<xz>"
  Bus Selector6/3 -> Subsystem4/3(vzk)  "<vz>"
  Bus Selector6/4 -> Subsystem4/4(vz)  "<vz>"
  Bus Selector4/3 -> Subsystem5/3(vxk)  "<vx>"
  Bus Selector4/2 -> Subsystem5/2(xx)  "<xx>"
  Bus Selector4/1 -> Subsystem5/1(xxk)  "<xx>"
  Bus Selector4/4 -> Subsystem5/4(vx)  "<vx>"
  Bus Selector5/1 -> Subsystem3/1(xyk)  "<xy>"
  Bus Selector5/2 -> Subsystem3/2(xy)  "<xy>"
  Bus Selector5/3 -> Subsystem3/3(vyk)  "<vy>"
  Bus Selector5/4 -> Subsystem3/4(vy)  "<vy>"
  Bus Creator2/1 -> Memory/1
  Subtract/1 -> Switch/2, Switch2/2
  L+B/1(u) -> MATLAB Function3/1(u)

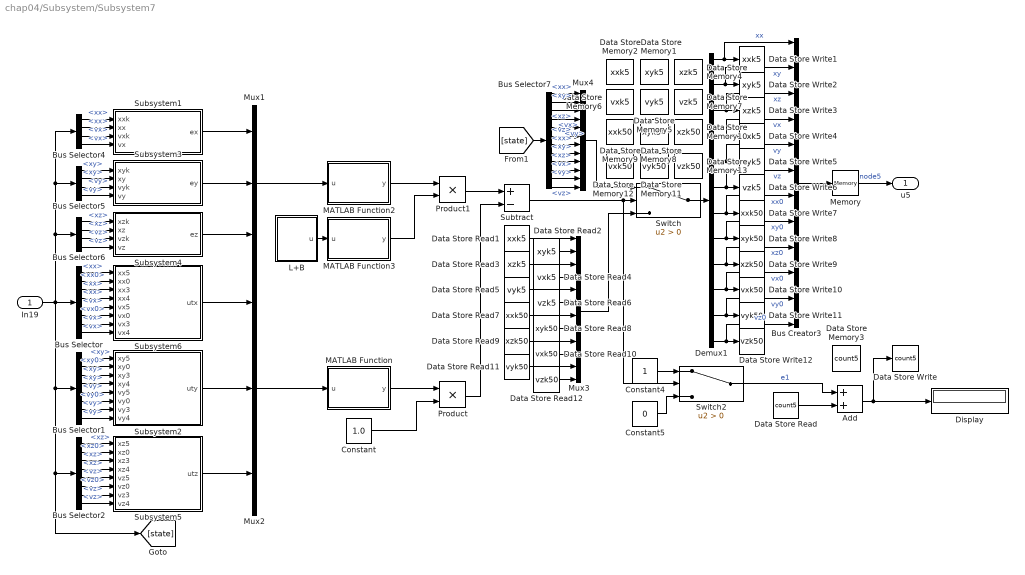
== system chap04/Subsystem/Subsystem7 ==
  In19 : Inport
  Add : Sum
  Bus Creator3 : BusCreator  Inputs=12
  Bus Selector : BusSelector  OutputSignals=state(tk).node5.xx,state(tk).node5.xx0,state(tk).node3.xx,state(tk).node4.xx,state(tk).node5.vx,state(tk).node5.vx0,state(tk).node3.vx,state(tk).node4.vx
  Bus Selector1 : BusSelector  OutputSignals=state(tk).node5.xy,state(tk).node5.xy0,state(tk).node3.xy,state(tk).node4.xy,state(tk).node5.vy,state(tk).node5.vy0,state(tk).node3.vy,state(tk).node4.vy
  Bus Selector2 : BusSelector  OutputSignals=state(tk).node5.xz,state(tk).node5.xz0,state(tk).node3.xz,state(tk).node4.xz,state(tk).node5.vz,state(tk).node5.vz0,state(tk).node3.vz,state(tk).node4.vz
  Bus Selector4 : BusSelector  OutputSignals=state(tk).node5.xx,state(t).node5.xx,state(tk).node5.vx,state(t).node5.vx
  Bus Selector5 : BusSelector  OutputSignals=state(tk).node5.xy,state(t).node5.xy,state(tk).node5.vy,state(t).node5.vy
  Bus Selector6 : BusSelector  OutputSignals=state(tk).node5.xz,state(t).node5.xz,state(tk).node5.vz,state(t).node5.vz
  Bus Selector7 : BusSelector  OutputSignals=state(t).node5.xx,state(t).node5.xy,state(t).node5.xz,state(t).node5.vx,state(t).node5.vy,state(t).node5.vz,state(t).node0.xx,state(t).node0.xy,state(t).node0.xz,state(t).node0.vx,state(t).node0.vy,state(t).node0.vz
  Constant : Constant  Value=1.0
  Constant4 : Constant
  Constant5 : Constant  Value=0
  Data Store Memory1 : DataStoreMemory  DataStoreName=xyk5  ReadBeforeWriteMsg=warning  WriteAfterWriteMsg=warning  WriteAfterReadMsg=warning  ShowAdditionalParam=off
  Data Store Memory10 : DataStoreMemory  DataStoreName=xzk50  ReadBeforeWriteMsg=warning  WriteAfterWriteMsg=warning  WriteAfterReadMsg=warning  ShowAdditionalParam=off
  Data Store Memory11 : DataStoreMemory  DataStoreName=vyk50  ReadBeforeWriteMsg=warning  WriteAfterWriteMsg=warning  WriteAfterReadMsg=warning  ShowAdditionalParam=off
  Data Store Memory12 : DataStoreMemory  DataStoreName=vxk50  ReadBeforeWriteMsg=warning  WriteAfterWriteMsg=warning  WriteAfterReadMsg=warning  ShowAdditionalParam=off
  Data Store Memory13 : DataStoreMemory  DataStoreName=vzk50  ReadBeforeWriteMsg=warning  WriteAfterWriteMsg=warning  WriteAfterReadMsg=warning  ShowAdditionalParam=off
  Data Store Memory2 : DataStoreMemory  DataStoreName=xxk5  ReadBeforeWriteMsg=warning  WriteAfterWriteMsg=warning  WriteAfterReadMsg=warning  ShowAdditionalParam=off
  Data Store Memory3 : DataStoreMemory  DataStoreName=count5  ReadBeforeWriteMsg=warning  WriteAfterWriteMsg=warning  WriteAfterReadMsg=warning  ShowAdditionalParam=off
  Data Store Memory4 : DataStoreMemory  DataStoreName=xzk5  ReadBeforeWriteMsg=warning  WriteAfterWriteMsg=warning  WriteAfterReadMsg=warning  ShowAdditionalParam=off
  Data Store Memory5 : DataStoreMemory  DataStoreName=vyk5  ReadBeforeWriteMsg=warning  WriteAfterWriteMsg=warning  WriteAfterReadMsg=warning  ShowAdditionalParam=off
  Data Store Memory6 : DataStoreMemory  DataStoreName=vxk5  ReadBeforeWriteMsg=warning  WriteAfterWriteMsg=warning  WriteAfterReadMsg=warning  ShowAdditionalParam=off
  Data Store Memory7 : DataStoreMemory  DataStoreName=vzk5  ReadBeforeWriteMsg=warning  WriteAfterWriteMsg=warning  WriteAfterReadMsg=warning  ShowAdditionalParam=off
  Data Store Memory8 : DataStoreMemory  DataStoreName=xyk50  ReadBeforeWriteMsg=warning  WriteAfterWriteMsg=warning  WriteAfterReadMsg=warning  ShowAdditionalParam=off
  Data Store Memory9 : DataStoreMemory  DataStoreName=xxk50  ReadBeforeWriteMsg=warning  WriteAfterWriteMsg=warning  WriteAfterReadMsg=warning  ShowAdditionalParam=off
  Data Store Read : DataStoreRead  DataStoreName=count5  IndexOptions=Index vector (dialog)  Indices=1  OutputSizes=1
  Data Store Read1 : DataStoreRead  DataStoreName=xxk5  IndexOptions=Index vector (dialog)  Indices=1  OutputSizes=1
  Data Store Read10 : DataStoreRead  DataStoreName=vxk50  IndexOptions=Index vector (dialog)  Indices=1  OutputSizes=1
  Data Store Read11 : DataStoreRead  DataStoreName=vyk50  IndexOptions=Index vector (dialog)  Indices=1  OutputSizes=1
  Data Store Read12 : DataStoreRead  DataStoreName=vzk50  IndexOptions=Index vector (dialog)  Indices=1  OutputSizes=1
  Data Store Read2 : DataStoreRead  DataStoreName=xyk5  IndexOptions=Index vector (dialog)  Indices=1  OutputSizes=1
  Data Store Read3 : DataStoreRead  DataStoreName=xzk5  IndexOptions=Index vector (dialog)  Indices=1  OutputSizes=1
  Data Store Read4 : DataStoreRead  DataStoreName=vxk5  IndexOptions=Index vector (dialog)  Indices=1  OutputSizes=1
  Data Store Read5 : DataStoreRead  DataStoreName=vyk5  IndexOptions=Index vector (dialog)  Indices=1  OutputSizes=1
  Data Store Read6 : DataStoreRead  DataStoreName=vzk5  IndexOptions=Index vector (dialog)  Indices=1  OutputSizes=1
  Data Store Read7 : DataStoreRead  DataStoreName=xxk50  IndexOptions=Index vector (dialog)  Indices=1  OutputSizes=1
  Data Store Read8 : DataStoreRead  DataStoreName=xyk50  IndexOptions=Index vector (dialog)  Indices=1  OutputSizes=1
  Data Store Read9 : DataStoreRead  DataStoreName=xzk50  IndexOptions=Index vector (dialog)  Indices=1  OutputSizes=1
  Data Store Write : DataStoreWrite  DataStoreName=count5  IndexOptions=Index vector (dialog)  Indices=1  OutputSizes=1
  Data Store Write1 : DataStoreWrite  DataStoreName=xxk5  IndexOptions=Index vector (dialog)  Indices=1  OutputSizes=1
  Data Store Write10 : DataStoreWrite  DataStoreName=vxk50  IndexOptions=Index vector (dialog)  Indices=1  OutputSizes=1
  Data Store Write11 : DataStoreWrite  DataStoreName=vyk50  IndexOptions=Index vector (dialog)  Indices=1  OutputSizes=1
  Data Store Write12 : DataStoreWrite  DataStoreName=vzk50  IndexOptions=Index vector (dialog)  Indices=1  OutputSizes=1
  Data Store Write2 : DataStoreWrite  DataStoreName=xyk5  IndexOptions=Index vector (dialog)  Indices=1  OutputSizes=1
  Data Store Write3 : DataStoreWrite  DataStoreName=xzk5  IndexOptions=Index vector (dialog)  Indices=1  OutputSizes=1
  Data Store Write4 : DataStoreWrite  DataStoreName=vxk5  IndexOptions=Index vector (dialog)  Indices=1  OutputSizes=1
  Data Store Write5 : DataStoreWrite  DataStoreName=vyk5  IndexOptions=Index vector (dialog)  Indices=1  OutputSizes=1
  Data Store Write6 : DataStoreWrite  DataStoreName=vzk5  IndexOptions=Index vector (dialog)  Indices=1  OutputSizes=1
  Data Store Write7 : DataStoreWrite  DataStoreName=xxk50  IndexOptions=Index vector (dialog)  Indices=1  OutputSizes=1
  Data Store Write8 : DataStoreWrite  DataStoreName=xyk50  IndexOptions=Index vector (dialog)  Indices=1  OutputSizes=1
  Data Store Write9 : DataStoreWrite  DataStoreName=xzk50  IndexOptions=Index vector (dialog)  Indices=1  OutputSizes=1
  Demux1 : Demux  Outputs=12
  Display : Display
  L+B : Subsystem
  MATLAB Function : MATLAB Function  TreatAsAtomicUnit=on
  MATLAB Function2 : MATLAB Function  TreatAsAtomicUnit=on
  MATLAB Function3 : MATLAB Function  TreatAsAtomicUnit=on
  Memory : Memory
  Mux1 : Mux  Inputs=3
  Mux2 : Mux  Inputs=3
  Mux3 : Mux  Inputs=12
  Mux4 : Mux  Inputs=12
  Product : Product
  Product1 : Product
  Subsystem1 : Subsystem
  Subsystem2 : Subsystem
  Subsystem3 : Subsystem
  Subsystem4 : Subsystem
  Subsystem5 : Subsystem
  Subsystem6 : Subsystem
  Subtract : Sum  Inputs=+-
  Switch : Switch  Criteria=u2 > Threshold
  Switch2 : Switch  Criteria=u2 > Threshold
  u5 : Outport
  wires:
  Bus Selector6/4 -> Subsystem4/4(vz)  "<vz>"
  Bus Selector6/3 -> Subsystem4/3(vzk)  "<vz>"
  Bus Selector6/2 -> Subsystem4/2(xz)  "<xz>"
  Bus Selector6/1 -> Subsystem4/1(xzk)  "<xz>"
  Bus Selector5/4 -> Subsystem3/4(vy)  "<vy>"
  Bus Selector5/3 -> Subsystem3/3(vyk)  "<vy>"
  Bus Selector5/2 -> Subsystem3/2(xy)  "<xy>"
  Bus Selector5/1 -> Subsystem3/1(xyk)  "<xy>"
  Bus Selector4/4 -> Subsystem1/4(vx)  "<vx>"
  Bus Selector4/3 -> Subsystem1/3(vxk)  "<vx>"
  Bus Selector4/2 -> Subsystem1/2(xx)  "<xx>"
  Bus Selector4/1 -> Subsystem1/1(xxk)  "<xx>"
  Memory/1 -> u5/1  "node5"
  Product/1 -> Subtract/2
  Switch2/1 -> Add/1  "e1"
  MATLAB Function3/1(y) -> Product1/2
  Constant5/1 -> Switch2/3
  Constant/1 -> Product/2
  Constant4/1 -> Switch2/1
  MATLAB Function2/1(y) -> Product1/1
  Mux1/1 -> MATLAB Function2/1(u)
  Subsystem4/1(ez) -> Mux1/3
  Subsystem1/1(ex) -> Mux1/1
  Add/1 -> Display/1, Data Store Write/1
  Product1/1 -> Subtract/1
  Mux2/1 -> MATLAB Function/1(u)
  MATLAB Function/1(y) -> Product/1
  Subsystem3/1(ey) -> Mux1/2
  Data Store Read/1 -> Add/2
  Subsystem2/1(uty) -> Mux2/2
  Subsystem6/1(utx) -> Mux2/1
  Subsystem5/1(utz) -> Mux2/3
  Subtract/1 -> Switch2/2, Switch/2
  Data Store Read7/1 -> Mux3/7
  Demux1/4 -> Data Store Write4/1, Bus Creator3/4  "vx"
  Demux1/10 -> Data Store Write10/1, Bus Creator3/10  "vx0"
  Bus Selector7/3 -> Mux4/3  "<xz>"
  Bus Selector7/9 -> Mux4/9  "<xz>"
  Bus Selector7/6 -> Mux4/6  "<vz>"
  Bus Selector7/4 -> Mux4/4  "<vx>"
  Bus Selector7/7 -> Mux4/7  "<xx>"
  Data Store Read12/1 -> Mux3/12
  Demux1/6 -> Data Store Write6/1, Bus Creator3/6  "vz"
  Bus Selector7/1 -> Mux4/1  "<xx>"
  Bus Selector7/8 -> Mux4/8  "<xy>"
  Data Store Read10/1 -> Mux3/10
  Mux3/1 -> Switch/3
  Demux1/12 -> Data Store Write12/1, Bus Creator3/12  "vz0"
  Demux1/7 -> Data Store Write7/1, Bus Creator3/7  "xx0"
  Bus Selector7/2 -> Mux4/2  "<xy>"
  Demux1/9 -> Data Store Write9/1, Bus Creator3/9  "xz0"
  Demux1/2 -> Data Store Write2/1, Bus Creator3/2  "xy"
  Demux1/5 -> Data Store Write5/1, Bus Creator3/5  "vy"
  Data Store Read8/1 -> Mux3/8
  Bus Creator3/1 -> Memory/1
  Demux1/8 -> Data Store Write8/1, Bus Creator3/8  "xy0"
  Data Store Read11/1 -> Mux3/11
  Data Store Read1/1 -> Mux3/1
  Demux1/1 -> Data Store Write1/1, Bus Creator3/1  "xx"
  Data Store Read2/1 -> Mux3/2
  Demux1/11 -> Data Store Write11/1, Bus Creator3/11  "vy0"
  Data Store Read9/1 -> Mux3/9
  Data Store Read4/1 -> Mux3/4
  Mux4/1 -> Switch/1
  Data Store Read3/1 -> Mux3/3
  Bus Selector7/5 -> Mux4/5  "<vy>"
  Data Store Read5/1 -> Mux3/5
  Data Store Read6/1 -> Mux3/6
  Demux1/3 -> Data Store Write3/1, Bus Creator3/3  "xz"
  Switch/1 -> Demux1/1
  [state] -> Bus Selector7/1
  Bus Selector7/10 -> Mux4/10  "<vx>"
  Bus Selector7/11 -> Mux4/11  "<vy>"
  Bus Selector7/12 -> Mux4/12  "<vz>"
  Bus Selector1/6 -> Subsystem2/6(vy0)  "<vy0>"
  Bus Selector1/7 -> Subsystem2/7(vy3)  "<vy>"
  Bus Selector/8 -> Subsystem6/8(vx4)  "<vx>"
  Bus Selector2/3 -> Subsystem5/3(xz3)  "<xz>"
  Bus Selector1/2 -> Subsystem2/2(xy0)  "<xy0>"
  Bus Selector/6 -> Subsystem6/6(vx0)  "<vx0>"
  Bus Selector2/1 -> Subsystem5/1(xz5)  "<xz>"
  Bus Selector2/5 -> Subsystem5/5(vz5)  "<vz>"
  Bus Selector2/2 -> Subsystem5/2(xz0)  "<xz0>"
  Bus Selector1/1 -> Subsystem2/1(xy5)  "<xy>"
  Bus Selector/1 -> Subsystem6/1(xx5)  "<xx>"
  Bus Selector2/4 -> Subsystem5/4(xz4)  "<xz>"
  Bus Selector1/3 -> Subsystem2/3(xy3)  "<xy>"
  Bus Selector/3 -> Subsystem6/3(xx3)  "<xx>"
  Bus Selector/2 -> Subsystem6/2(xx0)  "<xx0>"
  In19/1 -> Bus Selector/1, Bus Selector2/1, [state], Bus Selector1/1, Bus Selector4/1, Bus Selector5/1, Bus Selector6/1
  Bus Selector1/4 -> Subsystem2/4(xy4)  "<xy>"
  Bus Selector1/8 -> Subsystem2/8(vy4)  "<vy>"
  Bus Selector/7 -> Subsystem6/7(vx3)  "<vx>"
  Bus Selector/4 -> Subsystem6/4(xx4)  "<xx>"
  Bus Selector/5 -> Subsystem6/5(vx5)  "<vx>"
  Bus Selector1/5 -> Subsystem2/5(vy5)  "<vy>"
  Bus Selector2/8 -> Subsystem5/8(vz4)  "<vz>"
  Bus Selector2/7 -> Subsystem5/7(vz3)  "<vz>"
  Bus Selector2/6 -> Subsystem5/6(vz0)  "<vz0>"
  L+B/1(u) -> MATLAB Function3/1(u)
